simulink model "quadrotor_model"  (R2021b)
settings: Solver=VariableStepAuto  StartTime=0.0  StopTime=35  RelTol=1e-3
InitFcn:
  | Kp1=30*eye(3); Kw1=Kp1;
  | Kp2=600*eye(3); Kw2=Kp2;
  | Kp3=900*eye(3); Kw3=Kp3;
undefined symbols (not defined in the file or in its folder): iskew, matrix_A, quadrotor_controller, quadrotor_dynamics, rpy_rotation
libraries: robotcorelib x5, matrix_library x2
settings Model: Creator=lyuk  LastModifiedBy=lyuk

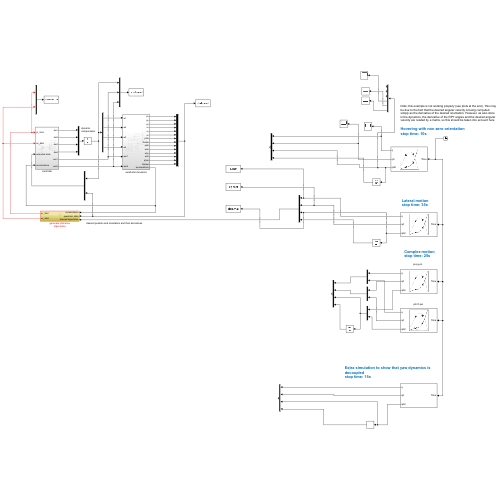
[thumbnail: Simulink's stored preview of the top-level diagram]
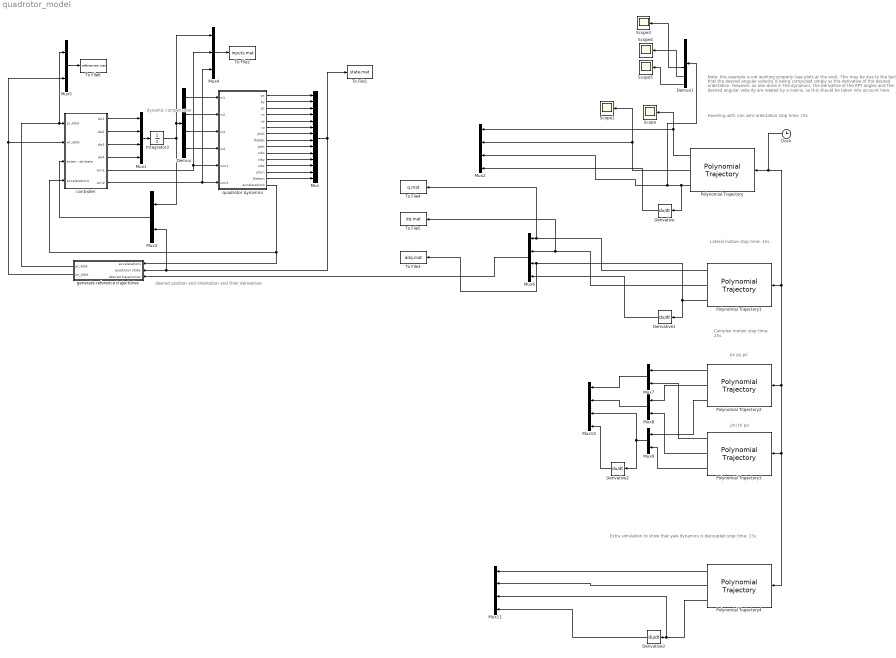
== system quadrotor_model ==
  note: Note: this example is not working properly (see plots at the end). This may be due to the fact that the desired angular velocity is being computed simply as the derivative of the desired orientation. However, as also done in the dynamics, the derivative of the RPY angles and the desired angular velocity are related by a matrix, so this should be taken into account here
  note: desired position and orientation and their derivatives
  note: px py pz
  note: Hovering with non zero orientation
      | stop time: 10s
  note: dynamic
      | compensator
  note: phi th psi
  note: Lateral motion
      | stop time: 35s
  note: Complex motion
      | stop time: 25s
  note: Extra simulation to show that yaw dynamics is decoupled
      | stop time: 15s
  Clock : Clock
  Demux : Demux
  Demux1 : Demux  Outputs=6
  Derivative{,1..3} (4 alike) : Derivative
  Integrator3 : Integrator  InitialCondition=ones(4,1)*613125/4
  Mux : Mux  Inputs=14
  Mux{1..2,6,10..11} (5 alike) : Mux
  Mux{3,5,7..9} (5 alike) : Mux  Inputs=2
  Mux4 : Mux  Inputs=3
  Polynomial Trajectory : robotcorelib/Polynomial Trajectory  WaypointSource=Internal  Waypoints=[zeros(3,11);0 deg2rad(10)*ones(1,4) zeros(1,6);zeros(1,3) deg2rad(-10)*ones(1,5) zeros(1,3);zeros(1,7) deg2rad(10)*ones(1,3) 0]  TimePoints=[1 1.5 2.5 3.4 3.5 4 5 5.9 6.5 7.5 8.2]  TimeInterval=[ 1, 4 ]  Method=Quintic Polynomial  ParameterSource=Internal  VelocityBoundaryCondition=zeros( 6, 11 )  AccelerationBoundaryCondition=zeros( 6, 11 )  SimulateUsing=Interpreted execution
  Polynomial Trajectory1 : robotcorelib/Polynomial Trajectory  WaypointSource=Internal  Waypoints=[0 5 5 5 5 0;0 0 0 5 5 0;zeros(4,6)]  TimePoints=[2 10 12 20 22 32]  TimeInterval=[ 1, 4 ]  Method=Quintic Polynomial  ParameterSource=Internal  VelocityBoundaryCondition=zeros( 6, 6 )  AccelerationBoundaryCondition=zeros( 6, 6 )  SimulateUsing=Interpreted execution
  Polynomial Trajectory2 : robotcorelib/Polynomial Trajectory  WaypointSource=Internal  Waypoints=[0 5 5 0;zeros(2,4)]  TimePoints=[2 10 13 22]  TimeInterval=[ 1, 4 ]  Method=Quintic Polynomial  ParameterSource=Internal  VelocityBoundaryCondition=zeros( 3, 4 )  AccelerationBoundaryCondition=zeros( 3, 4 )  SimulateUsing=Interpreted execution
  Polynomial Trajectory3 : robotcorelib/Polynomial Trajectory  WaypointSource=Internal  Waypoints=[zeros(1,6);0 -deg2rad(10) -deg2rad(10) deg2rad(10) deg2rad(10) 0;zeros(1,6)]  TimePoints=[2 3 12 13 23 24]  TimeInterval=[ 1, 4 ]  Method=Quintic Polynomial  ParameterSource=Internal  VelocityBoundaryCondition=zeros( 3, 6 )  AccelerationBoundaryCondition=zeros( 3, 6 )  SimulateUsing=Interpreted execution
  Polynomial Trajectory4 : robotcorelib/Polynomial Trajectory  WaypointSource=Internal  Waypoints=[zeros(4,8);zeros(1,4) 0 deg2rad(10) deg2rad(10) 0;0 deg2rad(10) deg2rad(10) 0 zeros(1,4)]  TimePoints=[1 2 4 5 6 7 9 10]  TimeInterval=[ 1, 4 ]  Method=Quintic Polynomial  ParameterSource=Internal  VelocityBoundaryCondition=zeros( 6, 8 )  AccelerationBoundaryCondition=zeros( 6, 8 )  SimulateUsing=Interpreted execution
  Scope{,1,3..5} (5 alike) : Scope
  To File1 : ToFile  Filename=state.mat  MatrixName=state
  To File2 : ToFile  Filename=inputs.mat  MatrixName=inputs
  To File3 : ToFile  Filename=ddq.mat  MatrixName=ddq
  To File4 : ToFile  Filename=q.mat  MatrixName=q
  To File5 : ToFile  Filename=dq.mat  MatrixName=dq
  To File6 : ToFile  Filename=references.mat  MatrixName=refs
  controller : Subsystem
  generate reference trajectories : Subsystem
  quadrotor dynamics : Subsystem
  wires:
  quadrotor dynamics/1(px) -> Mux/1
  quadrotor dynamics/2(py) -> Mux/2
  quadrotor dynamics/3(pz) -> Mux/3
  quadrotor dynamics/4(vx) -> Mux/4
  quadrotor dynamics/5(vy) -> Mux/5
  quadrotor dynamics/6(vz) -> Mux/6
  quadrotor dynamics/7(phib) -> Mux/7
  quadrotor dynamics/8(thetab) -> Mux/8
  quadrotor dynamics/9(psib) -> Mux/9
  quadrotor dynamics/10(wbx) -> Mux/10
  quadrotor dynamics/11(wby) -> Mux/11
  quadrotor dynamics/12(wbz) -> Mux/12
  quadrotor dynamics/13(phim) -> Mux/13
  quadrotor dynamics/14(thetam) -> Mux/14
  Mux/1 -> Mux3/2, generate reference trajectories/2(quadrotor state), To File1/1
  controller/5(wm1) -> Mux4/2, quadrotor dynamics/5(wm1)
  controller/6(wm2) -> Mux4/3, quadrotor dynamics/6(wm2)
  controller/1(dw1) -> Mux1/1
  controller/2(dw2) -> Mux1/2
  controller/3(dw3) -> Mux1/3
  controller/4(dw4) -> Mux1/4
  Mux1/1 -> Integrator3/1
  Integrator3/1 -> Mux3/1, Mux4/1, Demux/1
  Demux/1 -> quadrotor dynamics/1(w1)
  Demux/2 -> quadrotor dynamics/2(w2)
  Demux/3 -> quadrotor dynamics/3(w3)
  Demux/4 -> quadrotor dynamics/4(w4)
  Clock/1 -> Polynomial Trajectory/1, Polynomial Trajectory4/1, Polynomial Trajectory3/1, Polynomial Trajectory2/1, Polynomial Trajectory1/1
  Polynomial Trajectory/1 -> Scope/1, Mux2/1
  quadrotor dynamics/15(accelerations) -> controller/4(accelerations), generate reference trajectories/1(accelerations)
  Polynomial Trajectory/2 -> Scope1/1, Mux2/2
  Polynomial Trajectory/3 -> Derivative/1, Demux1/1, Mux2/3
  Derivative/1 -> Mux2/4
  generate reference trajectories/1(pr_3dot) -> Mux5/1, controller/1(pr_3dot)
  generate reference trajectories/2(wr_ddot) -> Mux5/2, controller/2(wr_ddot)
  Mux3/1 -> controller/3(extended state)
  Demux1/4 -> Scope3/1
  Demux1/5 -> Scope4/1
  Demux1/6 -> Scope5/1
  Polynomial Trajectory1/1 -> To File4/1, Mux6/1
  Polynomial Trajectory1/2 -> To File5/1, Mux6/2
  Polynomial Trajectory1/3 -> Derivative1/1, To File3/1, Mux6/3
  Derivative1/1 -> Mux6/4
  Polynomial Trajectory2/1 -> Mux7/1
  Polynomial Trajectory3/1 -> Mux7/2
  Polynomial Trajectory2/2 -> Mux8/1
  Polynomial Trajectory3/2 -> Mux8/2
  Polynomial Trajectory2/3 -> Mux9/1
  Polynomial Trajectory3/3 -> Mux9/2
  Mux9/1 -> Mux10/3, Derivative2/1
  Derivative2/1 -> Mux10/4
  Mux7/1 -> Mux10/1
  Mux8/1 -> Mux10/2
  Mux4/1 -> To File2/1
  Mux5/1 -> To File6/1
  Polynomial Trajectory4/3 -> Mux11/3, Derivative3/1
  Polynomial Trajectory4/1 -> Mux11/1
  Polynomial Trajectory4/2 -> Mux11/2
  Derivative3/1 -> Mux11/4
  Mux6/1 -> generate reference trajectories/3(desired trajectories)

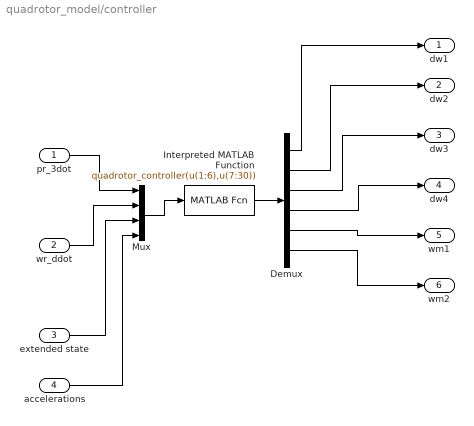
== system quadrotor_model/controller ==
  pr_3dot : Inport
  wr_ddot : Inport  Port=2
  extended state : Inport  Port=3
  accelerations : Inport  Port=4
  Demux : Demux  Outputs=6
  Interpreted MATLAB Function : MATLABFcn  MATLABFcn=quadrotor_controller(u(1:6),u(7:30))  OutputDimensions=[6,1]  OutputSignalType=real  Output1D=off
  Mux : Mux
  dw1 : Outport
  dw2 : Outport  Port=2
  dw3 : Outport  Port=3
  dw4 : Outport  Port=4
  wm1 : Outport  Port=5
  wm2 : Outport  Port=6
  wires:
  Mux/1 -> Interpreted MATLAB Function/1
  pr_3dot/1 -> Mux/1
  wr_ddot/1 -> Mux/2
  extended state/1 -> Mux/3
  Interpreted MATLAB Function/1 -> Demux/1
  Demux/1 -> dw1/1
  Demux/2 -> dw2/1
  Demux/3 -> dw3/1
  Demux/4 -> dw4/1
  Demux/5 -> wm1/1
  Demux/6 -> wm2/1
  accelerations/1 -> Mux/4

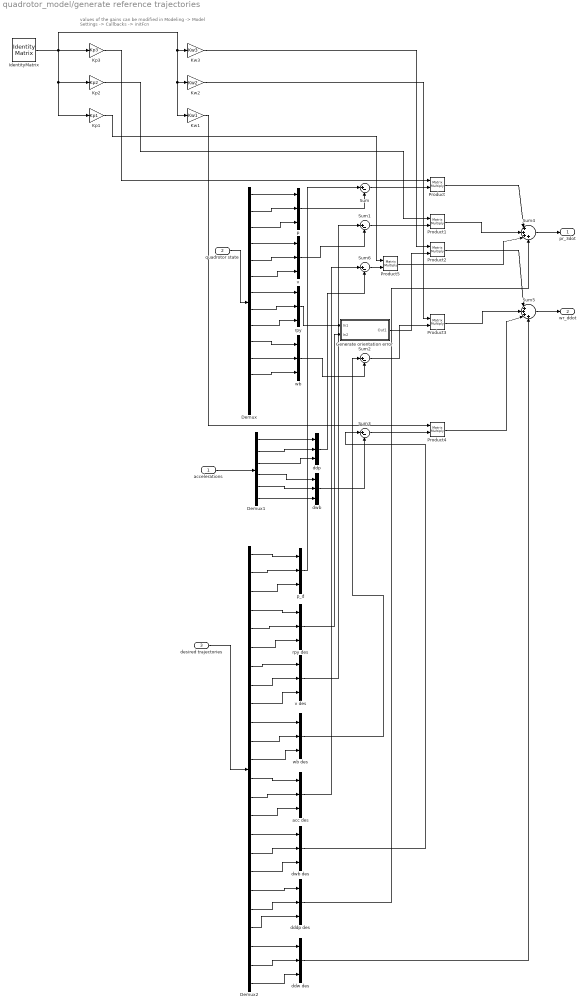
== system quadrotor_model/generate reference trajectories ==
  note: values of the gains can be modified in
      | Modeling -> Model Settings -> Callbacks -> initFcn
  accelerations : Inport
  quadrotor state : Inport  Port=2
  desired trajectories : Inport  Port=3
  Demux : Demux  Outputs=14
  Demux1 : Demux  Outputs=6
  Demux2 : Demux  Outputs=24
  Generate orientation error : Subsystem
  IdentityMatrix : IdentityMatrix  OutputDimensions=3
  Kp1 : Gain  Gain=Kp1
  Kp2 : Gain  Gain=Kp2
  Kp3 : Gain  Gain=Kp3
  Kw1 : Gain  Gain=Kw1
  Kw2 : Gain  Gain=Kw2
  Kw3 : Gain  Gain=Kw3
  Product{,1..5} (6 alike) : Product  Multiplication=Matrix(*)
  Sum{,1..3,6} (5 alike) : Sum  Inputs=|+-
  Sum4 : Sum  Inputs=|++++
  Sum5 : Sum  Inputs=|++++
  acc des : Mux  Inputs=3
  dddp des : Mux  Inputs=3
  ddp : Mux  Inputs=3
  ddw des : Mux  Inputs=3
  dwb : Mux  Inputs=3
  dwb des : Mux  Inputs=3
  p : Mux  Inputs=3
  p_d : Mux  Inputs=3
  rpy : Mux  Inputs=3
  rpy des : Mux  Inputs=3
  v : Mux  Inputs=3
  v des : Mux  Inputs=3
  wb : Mux  Inputs=3
  wb des : Mux  Inputs=3
  pr_3dot : Outport
  wr_ddot : Outport  Port=2
  wires:
  quadrotor state/1 -> Demux/1
  Demux/1 -> p/1
  Demux/2 -> p/2
  Demux/3 -> p/3
  p/1 -> Sum/2
  Sum/1 -> Product/2
  IdentityMatrix/1 -> Kp1/1, Kp2/1, Kw1/1, Kw2/1, Kw3/1, Kp3/1
  Kp3/1 -> Product/1
  Sum1/1 -> Product1/2
  v/1 -> Sum1/2
  Demux/6 -> v/3
  Demux/5 -> v/2
  Demux/4 -> v/1
  Kp2/1 -> Product1/1
  Demux/7 -> rpy/1
  Demux/8 -> rpy/2
  Demux/9 -> rpy/3
  rpy/1 -> Generate orientation error/1(In1)
  Generate orientation error/1(Out1) -> Product2/2
  Kw3/1 -> Product2/1
  Demux/12 -> wb/3
  Demux/11 -> wb/2
  Demux/10 -> wb/1
  wb/1 -> Sum2/2
  Sum2/1 -> Product3/2
  Kw2/1 -> Product3/1
  Sum3/1 -> Product4/2
  Kw1/1 -> Product4/1
  Sum4/1 -> pr_3dot/1
  Sum5/1 -> wr_ddot/1
  accelerations/1 -> Demux1/1
  Demux1/6 -> dwb/3
  Demux1/5 -> dwb/2
  Demux1/4 -> dwb/1
  dwb/1 -> Sum3/2
  Demux1/1 -> ddp/1
  Demux1/2 -> ddp/2
  Demux1/3 -> ddp/3
  desired trajectories/1 -> Demux2/1
  Demux2/1 -> p_d/1
  Demux2/2 -> p_d/2
  Demux2/3 -> p_d/3
  p_d/1 -> Sum/1
  Demux2/4 -> rpy des/1
  Demux2/5 -> rpy des/2
  Demux2/6 -> rpy des/3
  Demux2/7 -> v des/1
  Demux2/8 -> v des/2
  Demux2/9 -> v des/3
  Demux2/10 -> wb des/1
  Demux2/11 -> wb des/2
  Demux2/12 -> wb des/3
  Demux2/13 -> acc des/1
  Demux2/14 -> acc des/2
  Demux2/15 -> acc des/3
  Demux2/16 -> dwb des/1
  Demux2/17 -> dwb des/2
  Demux2/18 -> dwb des/3
  ddp/1 -> Sum6/2
  Sum6/1 -> Product5/2
  Kp1/1 -> Product5/1
  Product/1 -> Sum4/1
  Product1/1 -> Sum4/2
  Product5/1 -> Sum4/3
  Demux2/20 -> dddp des/2
  Demux2/19 -> dddp des/1
  Demux2/21 -> dddp des/3
  Demux2/22 -> ddw des/1
  Demux2/23 -> ddw des/2
  Demux2/24 -> ddw des/3
  dddp des/1 -> Sum4/4
  Product2/1 -> Sum5/1
  Product3/1 -> Sum5/2
  Product4/1 -> Sum5/3
  rpy des/1 -> Generate orientation error/2(In2)
  v des/1 -> Sum1/1
  acc des/1 -> Sum6/1
  dwb des/1 -> Sum3/1
  wb des/1 -> Sum2/1
  ddw des/1 -> Sum5/4

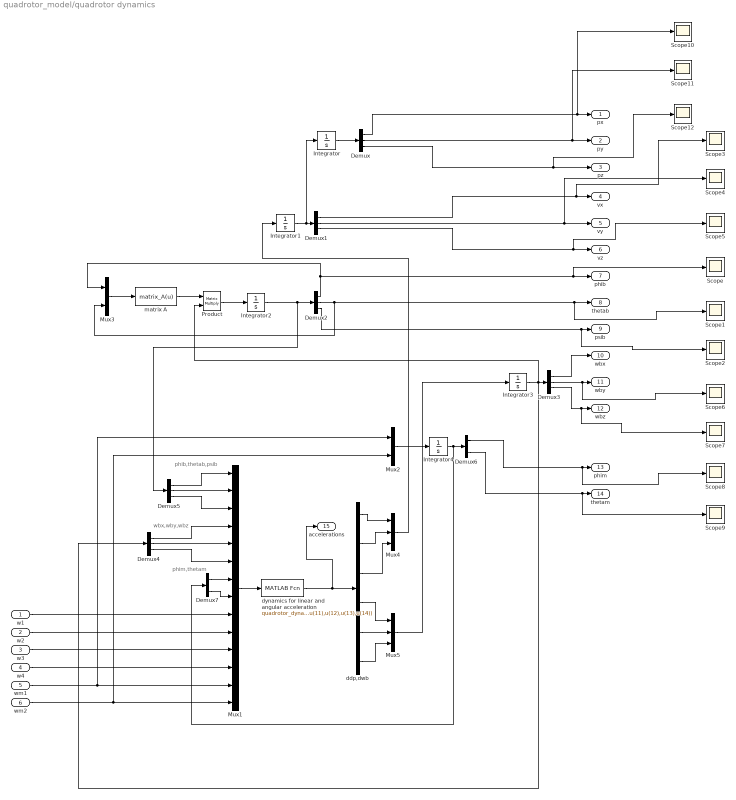
== system quadrotor_model/quadrotor dynamics ==
  note: phim,thetam
  note: wbx,wby,wbz
  note: phib,thetab,psib
  w1 : Inport
  w2 : Inport  Port=2
  w3 : Inport  Port=3
  w4 : Inport  Port=4
  wm1 : Inport  Port=5
  wm2 : Inport  Port=6
  Demux{,1..5} (6 alike) : Demux  Outputs=3
  Demux6 : Demux  Outputs=2
  Demux7 : Demux  Outputs=2
  Integrator{,1..3} (4 alike) : Integrator  InitialCondition=[0 0 0]'
  Integrator4 : Integrator  InitialCondition=[0 0]'
  Mux1 : Mux  Inputs=14
  Mux2 : Mux  Inputs=2
  Mux3 : Mux  Inputs=2
  Mux4 : Mux  Inputs=3
  Mux5 : Mux  Inputs=3
  Product : Product  Multiplication=Matrix(*)
  Scope{,1..12} (13 alike) : Scope
  ddp,dwb : Demux  Outputs=6
  dynamics for linear and angular acceleration : MATLABFcn  MATLABFcn=quadrotor_dynamics(u(1),u(2),u(3),u(4),u(5),u(6),u(7),u(8),u(9),u(10),u(11),u(12),u(13),u(14))  OutputDimensions=[6,1]  Output1D=off
  matrix A : MATLABFcn  MATLABFcn=matrix_A(u)  OutputDimensions=[3,3]  Output1D=off
  px : Outport
  py : Outport  Port=2
  pz : Outport  Port=3
  vx : Outport  Port=4
  vy : Outport  Port=5
  vz : Outport  Port=6
  phib : Outport  Port=7
  thetab : Outport  Port=8
  psib : Outport  Port=9
  wbx : Outport  Port=10
  wby : Outport  Port=11
  wbz : Outport  Port=12
  phim : Outport  Port=13
  thetam : Outport  Port=14
  accelerations : Outport  Port=15
  wires:
  Integrator1/1 -> Integrator/1, Demux1/1
  Demux/1 -> Scope10/1, px/1
  Demux/2 -> Scope11/1, py/1
  Demux/3 -> Scope12/1, pz/1
  Integrator/1 -> Demux/1
  Demux1/1 -> Scope3/1, vx/1
  Demux1/2 -> vy/1, Scope4/1
  Demux1/3 -> Scope5/1, vz/1
  Integrator2/1 -> Demux5/1, Demux2/1
  Demux2/1 -> Scope/1, phib/1, Mux3/1
  Demux2/2 -> Mux3/2, Scope1/1, thetab/1
  Demux2/3 -> Scope2/1, psib/1
  Mux1/1 -> dynamics for linear and angular acceleration/1
  Integrator3/1 -> Demux4/1, Product/2, Demux3/1
  Demux3/1 -> wbx/1
  Demux3/2 -> Scope6/1, wby/1
  Demux3/3 -> Scope7/1, wbz/1
  ddp,dwb/1 -> Mux4/1
  Demux4/1 -> Mux1/4
  Demux4/2 -> Mux1/5
  Demux4/3 -> Mux1/6
  Demux5/2 -> Mux1/2
  Demux5/1 -> Mux1/1
  Demux5/3 -> Mux1/3
  w1/1 -> Mux1/9
  w2/1 -> Mux1/10
  wm2/1 -> Mux1/14, Mux2/2
  wm1/1 -> Mux2/1, Mux1/13
  w4/1 -> Mux1/12
  w3/1 -> Mux1/11
  Integrator4/1 -> Demux7/1, Demux6/1
  Demux6/1 -> Scope8/1, phim/1
  Demux6/2 -> Scope9/1, thetam/1
  Mux2/1 -> Integrator4/1
  Demux7/1 -> Mux1/7
  Demux7/2 -> Mux1/8
  Product/1 -> Integrator2/1
  Mux3/1 -> matrix A/1
  matrix A/1 -> Product/1
  ddp,dwb/2 -> Mux4/2
  ddp,dwb/3 -> Mux4/3
  ddp,dwb/5 -> Mux5/2
  ddp,dwb/4 -> Mux5/1
  ddp,dwb/6 -> Mux5/3
  Mux5/1 -> Integrator3/1
  Mux4/1 -> Integrator1/1
  dynamics for linear and angular acceleration/1 -> accelerations/1, ddp,dwb/1

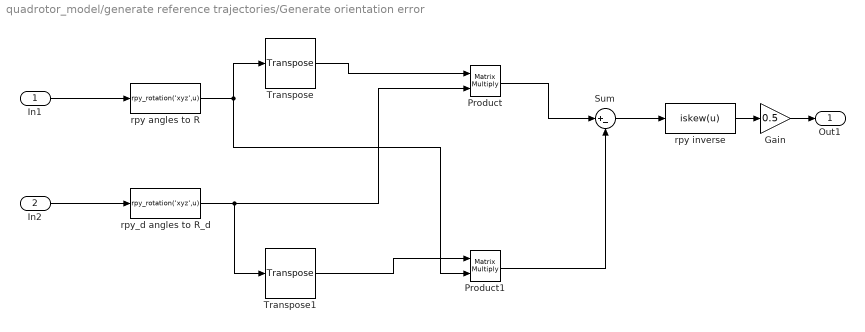
== system quadrotor_model/generate reference trajectories/Generate orientation error ==
  In1 : Inport
  In2 : Inport  Port=2
  Gain : Gain  Gain=0.5
  Product : Product  Multiplication=Matrix(*)
  Product1 : Product  Multiplication=Matrix(*)
  Sum : Sum  Inputs=|+-
  Transpose : matrix_library/Transpose
      settings: SourceProductBaseCode=SL
  Transpose1 : matrix_library/Transpose
      settings: SourceProductBaseCode=SL
  rpy angles to R : MATLABFcn  MATLABFcn=rpy_rotation('xyz',u)  OutputDimensions=[3,3]  Output1D=off
  rpy inverse : MATLABFcn  MATLABFcn=iskew(u)  OutputDimensions=[3,1]  Output1D=off
  rpy_d angles to R_d : MATLABFcn  MATLABFcn=rpy_rotation('xyz',u)  OutputDimensions=[3,3]  Output1D=off
  Out1 : Outport
  wires:
  In1/1 -> rpy angles to R/1
  In2/1 -> rpy_d angles to R_d/1
  rpy angles to R/1 -> Product1/2, Transpose/1
  Transpose/1 -> Product/1
  rpy_d angles to R_d/1 -> Transpose1/1, Product/2
  Transpose1/1 -> Product1/1
  Product/1 -> Sum/1
  Product1/1 -> Sum/2
  Sum/1 -> rpy inverse/1
  rpy inverse/1 -> Gain/1
  Gain/1 -> Out1/1
